simulink model "lab7"  (R2021b)
settings: Solver=FixedStepAuto  StartTime=0.0  StopTime=180  FixedStep=0.001  RelTol=1e-3
model workspace (MAT data in the model file):
  Ti = 200
values from neighbouring files (symbols this model uses):
  ddMax = 3    [sysdata.m]
  deltaMax = 30    [sysdata.m]
  fConst = 0    [sysdata.m]
  K = 0.08    [sysdata.m]
  Kaw = 1    [sysdata.m]
  Kc = 0.7045    [sysdata.m]
  phiZad = 30    [sysdata.m]
  T = aT(i)    [lab7go.m]    (also in sysdata.m = 1)
  Toc = 5    [sysdata.m]
  Tr = 1    [sysdata.m]
  Ts = 18    [sysdata.m]
undefined symbols (not defined in the file or in its folder): dD, nD
settings Model: Creator=valeria  LastModifiedBy=Ivan
settings SolverCC: AlgebraicLoopSolver=TrustRegion
settings DebuggingCC: SFMachineParentedDataDiag=warning

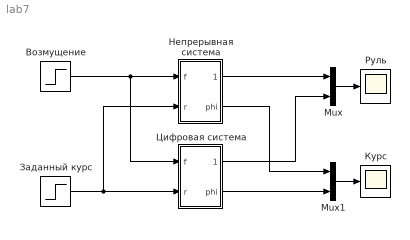
== system lab7 ==
  Mux : Mux  Inputs=2
  Mux1 : Mux  Inputs=2
  Возмущение : Step  Time=0  After=fConst  SampleTime=0
  Заданный курс : Step  Time=0  After=phiZad  SampleTime=0
  Курс : Scope
  Непрерывная система : Subsystem
  Руль : Scope
  Цифровая система : Subsystem
  wires:
  Возмущение/1 -> Цифровая система/1(f), Непрерывная система/1(f)
  Mux/1 -> Руль/1
  Mux1/1 -> Курс/1
  Непрерывная система/1(delta) -> Mux/1
  Непрерывная система/2(phi) -> Mux1/1
  Заданный курс/1 -> Цифровая система/2(r), Непрерывная система/2(r)
  Цифровая система/1(delta) -> Mux/2
  Цифровая система/2(phi) -> Mux1/2

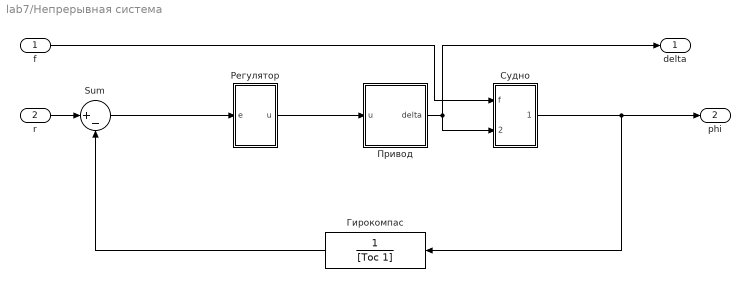
== system lab7/Непрерывная система ==
  f : Inport
  r : Inport  Port=2
  " Гирокомпас" : TransferFcn  Denominator=[Toc 1]
  Sum : Sum  Inputs=|+-
  Привод : Subsystem
  Регулятор : Subsystem
  Судно : Subsystem
  delta : Outport
  phi : Outport  Port=2
  wires:
  r/1 -> Sum/1
  Судно/1(phi) -> phi/1, " Гирокомпас"/1
  " Гирокомпас"/1 -> Sum/2
  Привод/1(delta) -> delta/1, Судно/2(delta)
  f/1 -> Судно/1(f)
  Sum/1 -> Регулятор/1(e)
  Регулятор/1(u) -> Привод/1(u)

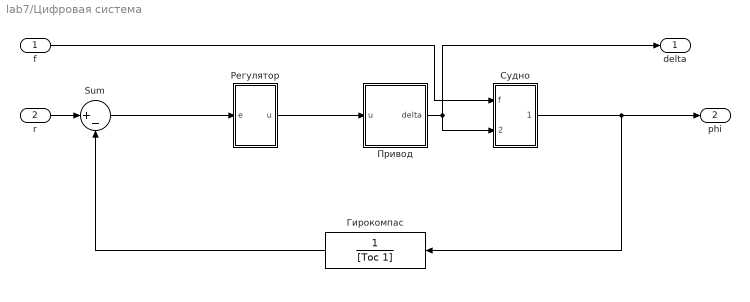
== system lab7/Цифровая система ==
  f : Inport
  r : Inport  Port=2
  " Гирокомпас" : TransferFcn  Denominator=[Toc 1]
  Sum : Sum  Inputs=|+-
  Привод : Subsystem
  Регулятор : Subsystem
  Судно : Subsystem
  delta : Outport
  phi : Outport  Port=2
  wires:
  r/1 -> Sum/1
  Судно/1(phi) -> phi/1, " Гирокомпас"/1
  " Гирокомпас"/1 -> Sum/2
  Привод/1(delta) -> delta/1, Судно/2(delta)
  f/1 -> Судно/1(f)
  Sum/1 -> Регулятор/1(e)
  Регулятор/1(u) -> Привод/1(u)

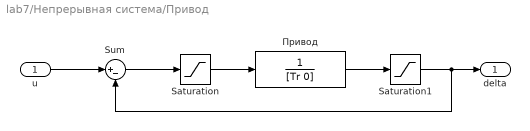
== system lab7/Непрерывная система/Привод ==
  u : Inport
  Saturation : Saturate  UpperLimit=+ddMax  LowerLimit=-ddMax
  Saturation1 : Saturate  UpperLimit=+deltaMax  LowerLimit=-deltaMax
  Sum : Sum  Inputs=|+-
  Привод : TransferFcn  Denominator=[Tr 0]
  delta : Outport
  wires:
  u/1 -> Sum/1
  Sum/1 -> Saturation/1
  Saturation/1 -> Привод/1
  Привод/1 -> Saturation1/1
  Saturation1/1 -> Sum/2, delta/1

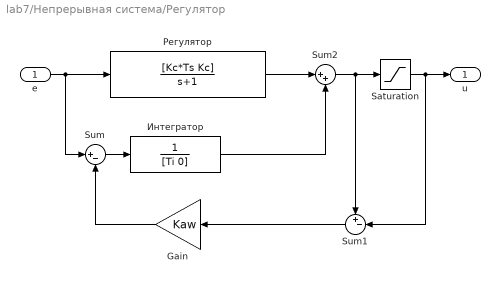
== system lab7/Непрерывная система/Регулятор ==
  e : Inport
  " Интегратор" : TransferFcn  Denominator=[Ti 0]
  Gain : Gain  Gain=Kaw
  Saturation : Saturate  UpperLimit=180  LowerLimit=-180
  Sum : Sum  Inputs=|+-
  Sum1 : Sum  Inputs=+-|
  Sum2 : Sum  Inputs=|++
  Регулятор : TransferFcn  Numerator=[Kc*Ts Kc]  Denominator=[1 1]
  u : Outport
  wires:
  " Интегратор"/1 -> Sum2/2
  e/1 -> Регулятор/1, Sum/1
  Регулятор/1 -> Sum2/1
  Sum2/1 -> Saturation/1, Sum1/1
  Sum/1 -> " Интегратор"/1
  Saturation/1 -> Sum1/2, u/1
  Sum1/1 -> Gain/1
  Gain/1 -> Sum/2

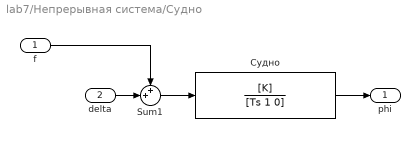
== system lab7/Непрерывная система/Судно ==
  f : Inport
  delta : Inport  Port=2
  Sum1 : Sum  Inputs=++|
  Судно : TransferFcn  Numerator=[K]  Denominator=[Ts 1 0]
  phi : Outport
  wires:
  Sum1/1 -> Судно/1
  Судно/1 -> phi/1
  delta/1 -> Sum1/2
  f/1 -> Sum1/1

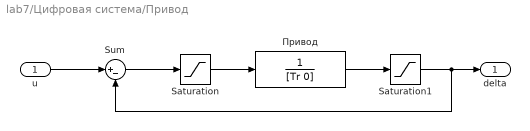
== system lab7/Цифровая система/Привод ==
  u : Inport
  Saturation : Saturate  UpperLimit=+ddMax  LowerLimit=-ddMax
  Saturation1 : Saturate  UpperLimit=+deltaMax  LowerLimit=-deltaMax
  Sum : Sum  Inputs=|+-
  Привод : TransferFcn  Denominator=[Tr 0]
  delta : Outport
  wires:
  u/1 -> Sum/1
  Sum/1 -> Saturation/1
  Saturation/1 -> Привод/1
  Привод/1 -> Saturation1/1
  Saturation1/1 -> Sum/2, delta/1

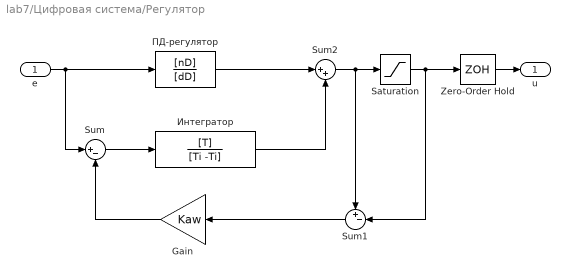
== system lab7/Цифровая система/Регулятор ==
  e : Inport
  Gain : Gain  Gain=Kaw
  Saturation : Saturate  UpperLimit=180  LowerLimit=-180
  Sum : Sum  Inputs=|+-
  Sum1 : Sum  Inputs=+-|
  Sum2 : Sum  Inputs=|++
  Zero-Order Hold : ZeroOrderHold  SampleTime=T
  Интегратор : DiscreteTransferFcn  Numerator=[T]  Denominator=[Ti -Ti]  SampleTime=T
  ПД-регулятор : DiscreteTransferFcn  Numerator=[nD]  Denominator=[dD]  SampleTime=T
  u : Outport
  wires:
  e/1 -> ПД-регулятор/1, Sum/1
  Sum2/1 -> Saturation/1, Sum1/1
  Saturation/1 -> Zero-Order Hold/1, Sum1/2
  Sum1/1 -> Gain/1
  Gain/1 -> Sum/2
  ПД-регулятор/1 -> Sum2/1
  Интегратор/1 -> Sum2/2
  Sum/1 -> Интегратор/1
  Zero-Order Hold/1 -> u/1

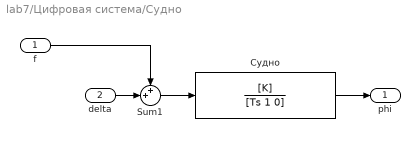
== system lab7/Цифровая система/Судно ==
  f : Inport
  delta : Inport  Port=2
  Sum1 : Sum  Inputs=++|
  Судно : TransferFcn  Numerator=[K]  Denominator=[Ts 1 0]
  phi : Outport
  wires:
  Sum1/1 -> Судно/1
  Судно/1 -> phi/1
  delta/1 -> Sum1/2
  f/1 -> Sum1/1
